simulink model "SerialCommunication"  (R2022a)
settings: Solver=FixedStepAuto  StartTime=0.0  StopTime=inf  RelTol=1e-3  EnableMultiTasking=on
libraries: svdutilitieslib x1, mbedblockslib x1
settings Model: ExtModeTrigDuration=10  Creator=adlipke  LastModifiedBy=adlipke
settings OptimizationCC: EnhancedBackFolding=on  PassReuseOutputArgsAs=Individual arguments  ZeroExternalMemoryAtStartup=off  ZeroInternalMemoryAtStartup=off  MaxStackSize=64  OptimizeBlockOrder=speed  DifferentSizesBufferReuse=on  OptimizationCustomize=off  EfficientTunableParamExpr=on
settings DebuggingCC: ParameterTunabilityLossMsg=error
settings HardwareCC: ProdBitPerPointer=32  ProdBitPerSizeT=32  ProdBitPerPtrDiffT=32  ProdLargestAtomicInteger=Long  ProdLargestAtomicFloat=Double  ProdWordSize=32  ProdLongLongMode=on  ProdHWDeviceType=ARM Compatible->ARM Cortex
settings SFSimCC: MATLABDynamicMemAlloc=off
settings RTWCC: SystemTargetFile=ert.tlc  HardwareBoard=STM32 Nucleo L476RG  TemplateMakefile=ert_default_tmf  Toolchain=GNU Tools for ARM Embedded Processors
settings CodeAppCC: ForceParamTrailComments=on  IgnoreCustomStorageClasses=off  OperatorAnnotations=on  SimulinkDataObjDesc=on  SFDataObjDesc=on  InsertBlockDesc=on
settings ERTTargetCC: ExtModeTransport=3  ExtModeStaticAlloc=on  ExtModeStaticAllocSize=2000  ExtModeMexFile=ext_xcp  ExtModeIntrfLevel=Level2 - Open

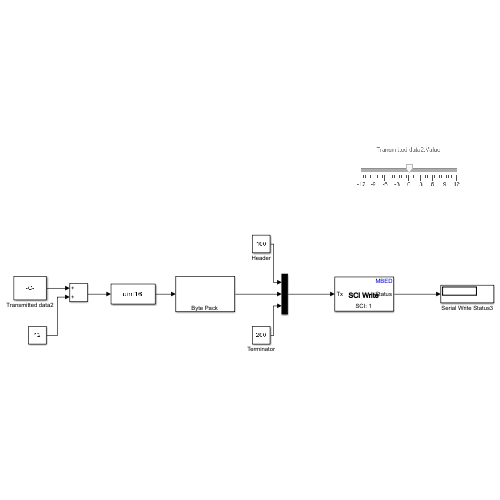
[thumbnail: Simulink's stored preview of the top-level diagram]
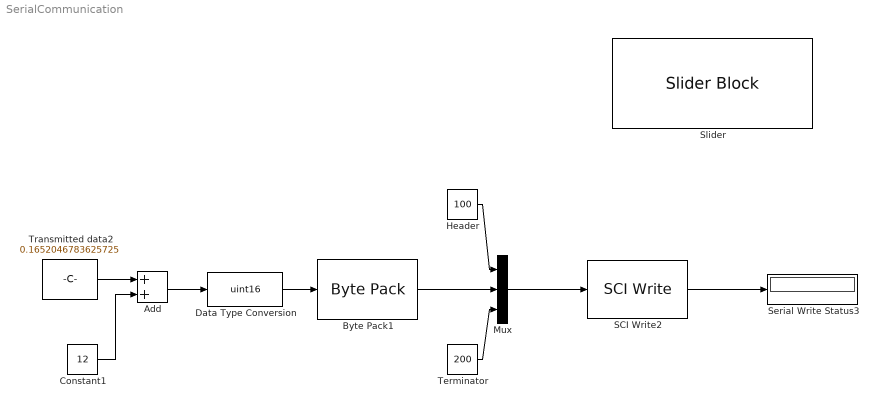
== system SerialCommunication ==
  Add : Sum  AccumDataTypeStr=uint16  OutDataTypeStr=uint16
  Byte Pack1 : svdutilitieslib/Byte Pack  maskPackedDataType=uint8  datatypes={'uint16'}  byteAlign=1  blockPlatform=arduinoert
      settings: SourceProductBaseCode=ANDROID,ARDUINO,ML_ARDUINO,ECCORTEXA,ECCORTEXR,SC_BEAGLEBONE_BLUE,EC_FREEDOM_BOARD,EC_FRDM_K64F,INTEL_BLOCKSET,MICROBIT,NUCLEO,NVIDIA,PX4AUTOPILOTS,RASPPIIO,STMICRODIS,TIC2000,XILINX_BLOCKSET
  Constant1 : Constant  Value=12  OutDataTypeStr=single
  Data Type Conversion : DataTypeConversion  OutDataTypeStr=uint16  SaturateOnIntegerOverflow=off  RndMeth=Floor
  Header : Constant  Value=100  OutDataTypeStr=uint8  SampleTime=0.01
  Mux : Mux  Inputs=3
  SCI Write2 : mbedblockslib/SCI Write  SCIModule=1  Baudrate=uint32(9600)  Parity=None  StopBits=1  HardwareFlowControl=None  ByteOrder=LittleEndian  OutputStatus=on
      settings: SourceProductBaseCode=MICROBIT,NUCLEO,STMICRODIS
  Serial Write Status3 : Display
  Slider : SliderBlock  ScaleMin=-12  ScaleMax=12
  Terminator : Constant  Value=200  OutDataTypeStr=uint8  SampleTime=0.01
  Transmitted data2 : Constant  Value=0.1652046783625725  OutDataTypeStr=single  SampleTime=0.01
  wires:
  Add/1 -> Data Type Conversion/1
  Data Type Conversion/1 -> Byte Pack1/1
  Terminator/1 -> Mux/3
  Constant1/1 -> Add/2
  Transmitted data2/1 -> Add/1
  Header/1 -> Mux/1
  Byte Pack1/1 -> Mux/2
  Mux/1 -> SCI Write2/1
  SCI Write2/1 -> Serial Write Status3/1
